simulink model "Active_Suspension_Control_Simulink"  (R2023b)
settings: Solver=VariableStepAuto  StartTime=0.0  StopTime=10.0  MaxStep=1e-3  RelTol=1e-3
values from neighbouring files (symbols this model uses):
  a = [1 20 3486.66666667 10555.5555556 168888.888889]    [Fuzzy_Workspace.mat]    (also in quarter_car_model.m = 0.8)
  b = [0 0 0.00333333333333 10555.6111112 168900.333335]    [Fuzzy_Workspace.mat]
  c_car = 1000    [Active_Suspension_Control.m]    (also in Fuzzy_Workspace.mat)
  k_car = 16000    [Active_Suspension_Control.m]    (also in Fuzzy_Workspace.mat)
  k_wheel = 190000    [Active_Suspension_Control.m]    (also in Fuzzy_Workspace.mat)
  m_car = 300    [Active_Suspension_Control.m]    (also in Fuzzy_Workspace.mat)
  m_wheel = 60    [Active_Suspension_Control.m]    (also in Fuzzy_Workspace.mat)
libraries: slpidlib x1
settings Model: Creator=hkurt  LastModifiedBy=hkurt

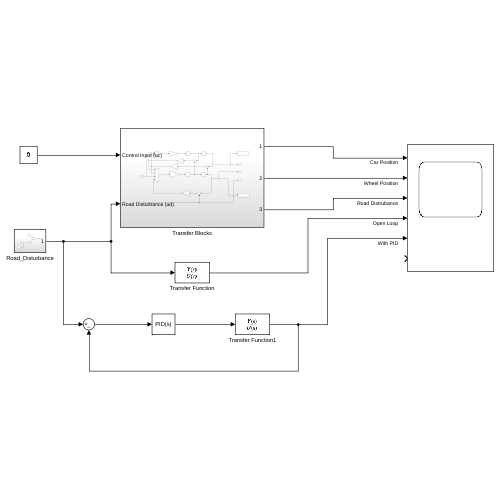
[thumbnail: Simulink's stored preview of the top-level diagram]
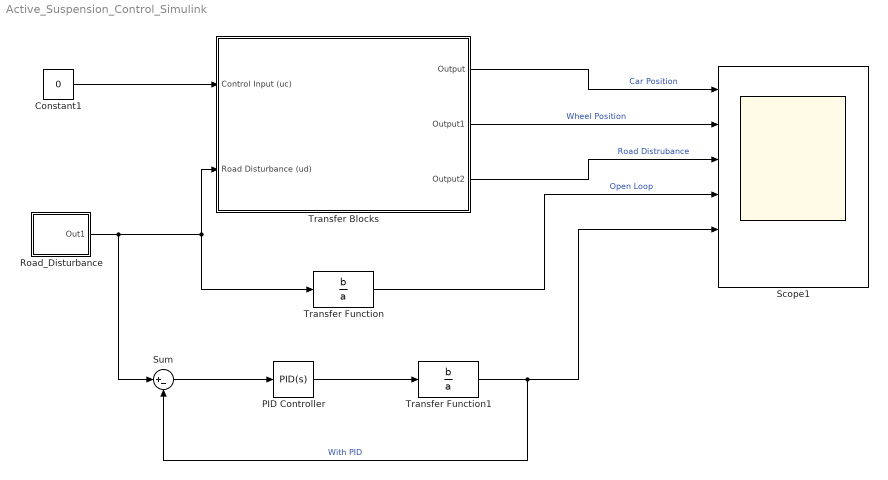
== system Active_Suspension_Control_Simulink ==
  Constant1 : Constant  Value=0
  PID Controller : slpidlib/PID Controller  Controller=PID  Form=Parallel  TimeDomain=Continuous-time  UseExternalTs=off  SampleTime=-1  IntegratorMethod=Forward Euler  FilterMethod=Forward Euler  ControllerParametersSource=internal  P=1  I=10  UseKiTs=off  D=0  N=100  UseFilter=on  TunerSelectOption=Transfer Function Based (PID Tuner App)  InitialConditionSource=internal  InitialConditionForIntegrator=0  InitialConditionForFilter=0  DifferentiatorICPrevScaledInput=0  ExternalReset=none  TrackingMode=off  Kt=1  LimitOutput=off  SatLimitsSource=internal  UpperSaturationLimit=inf  LowerSaturationLimit=-inf  LinearizeAsGain=on  AntiWindupMode=none  Kb=1  LimitIntegrator=off  UpperIntegratorSaturationLimit=inf  LowerIntegratorSaturationLimit=-inf  POutMin=[]  POutMax=[]  IOutMin=[]  IOutMax=[]  DOutMin=[]  DOutMax=[]  NOutMin=[]  NOutMax=[]  SumOutMin=[]  SumOutMax=[]  SaturationOutMin=[]  SaturationOutMax=[]  PParamMin=[]  PParamMax=[]  IParamMin=[]  IParamMax=[]  DParamMin=[]  DParamMax=[]  NParamMin=[]  NParamMax=[]  KbParamMin=[]  KbParamMax=[]  KtParamMin=[]  KtParamMax=[]  KbOutMin=[]  KbOutMax=[]  KtOutMin=[]  KtOutMax=[]  IntegratorOutMin=[]  IntegratorOutMax=[]  FilterOutMin=[]  FilterOutMax=[]  SumI1OutMin=[]  SumI1OutMax=[]  SumI2OutMin=[]  SumI2OutMax=[]  SumI3OutMin=[]  SumI3OutMax=[]  SumI4OutMin=[]  SumI4OutMax=[]  SumDOutMin=[]  SumDOutMax=[]  DifferentiatorOutMin=[]  DifferentiatorOutMax=[]  FilterDiffOutCoefMin=[]  FilterDiffOutCoefMax=[]  ReciprocalOutMin=[]  ReciprocalOutMax=[]  SumDenOutMin=[]  SumDenOutMax=[]  SumNumOutMin=[]  SumNumOutMax=[]  DivideOutMin=[]  DivideOutMax=[]  UdiffTsProdOutMin=[]  UdiffTsProdOutMax=[]  NTsProdOutMin=[]  NTsProdOutMax=[]  UintegralTsProdOutMin=[]  UintegralTsProdOutMax=[]  UngainTsProdOutMin=[]  UngainTsProdOutMax=[]  ClampingZeroOutDataTypeStr=Inherit: Inherit via back propagation  ClampingZeroOutMin=[]  ClampingZeroOutMax=[]  FilterDenConstantOutDataTypeStr=Inherit: Inherit via back propagation  FilterDenConstantOutMin=[]  FilterDenConstantOutMax=[]  PCopyOutDataTypeStr=Inherit: Inherit via back propagation  PCopyOutMin=[]  PCopyOutMax=[]  NCopyOutDataTypeStr=Inherit: Inherit via back propagation  NCopyOutMin=[]  NCopyOutMax=[]  IntegratorContinuousStateAttributes=''  IntegratorStateMustResolveToSignalObject=off  IntegratorRTWStateStorageClass=Auto  FilterContinuousStateAttributes=''  FilterStateMustResolveToSignalObject=off  FilterRTWStateStorageClass=Auto  ParallelPVariant=InternalParameters  IdealPVariant=Disabled  IVariant=InternalParameters  DVariant=InternalParameters  IntegratorVariant=Continuous  SatVariant=Disabled  AWVariant=Passthrough  PCopyVariant=Disabled  TRVariant=Disabled  FdbkBlocksVariant=Forward  IdealPFdbkVariant=Disabled  SatFdbkVariant=Disabled  DerivativeFilterVariant=ContFilter  NVariant=InternalParameters  NCopyVariant=Disabled  FilterICVariant=InternalICsFilter  IntegratorICVariant=InternalICs  ExternalResetVariant=Disabled  TRSumVariant=Passthrough  SumFdbkVariant=Disabled  SumVariant=Sum_PID  TsampFilterVariant=InternalTs  TsampNgainVariant=Passthrough  TsampIntegralVariant=Disabled_SignalSpec  ExternalSaturationOutDataTypeStr=Inherit: Same as second input
  Road_Disturbance : Subsystem
  Scope1 : Scope  NumInputPorts=6
  Sum : Sum  Inputs=|+-
  Transfer Blocks : Subsystem
  Transfer Function : TransferFcn  Numerator=b  Denominator=a
  Transfer Function1 : TransferFcn  Numerator=b  Denominator=a
  wires:
  Transfer Blocks/2(Output1) -> Scope1/2  "Wheel Position"
  Transfer Blocks/3(Output2) -> Scope1/3  "Road Distrubance"
  Constant1/1 -> Transfer Blocks/1(Control Input (uc))
  Transfer Blocks/1(Output) -> Scope1/1  "Car Position"
  Road_Disturbance/1(Out1) -> Sum/1, Transfer Function/1, Transfer Blocks/2(Road Disturbance (ud))
  Transfer Function/1 -> Scope1/4  "Open Loop"
  PID Controller/1 -> Transfer Function1/1
  Transfer Function1/1 -> Scope1/5, Sum/2  "With PID"
  Sum/1 -> PID Controller/1

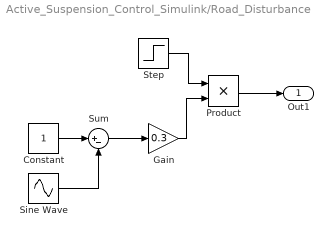
== system Active_Suspension_Control_Simulink/Road_Disturbance ==
  Constant : Constant
  Gain : Gain  Gain=0.3
  Product : Product
  Sine Wave : Sin  Frequency=2*pi  Phase=pi/2  SampleTime=0
  Step : Step  Before=1  After=0  SampleTime=0
  Sum : Sum  Inputs=|+-
  Out1 : Outport
  wires:
  Constant/1 -> Sum/1
  Step/1 -> Product/1
  Sum/1 -> Gain/1
  Gain/1 -> Product/2
  Product/1 -> Out1/1
  Sine Wave/1 -> Sum/2

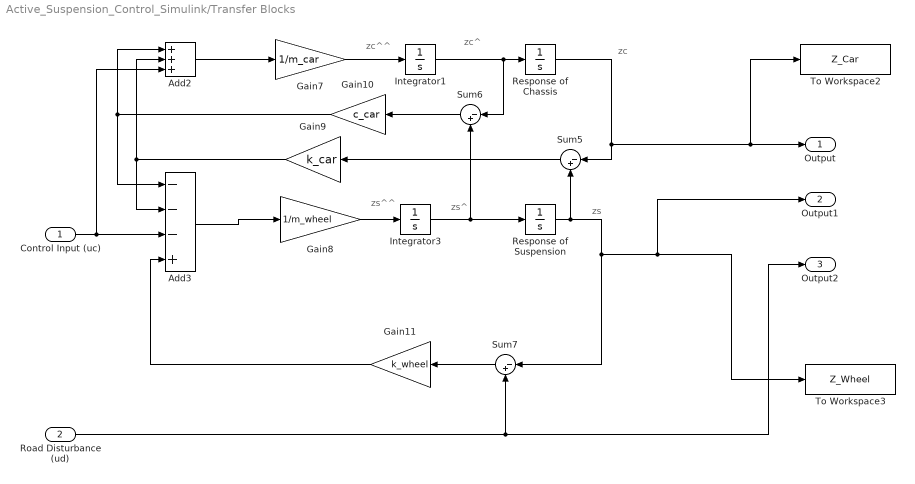
== system Active_Suspension_Control_Simulink/Transfer Blocks ==
  note: zs
  note: zc^^
  note: zc
  note: zc^
  note: zs^^
  note: zs^
  Control Input (uc) : Inport
  Road Disturbance (ud) : Inport  Port=2
  Add2 : Sum  Inputs=+++
  Add3 : Sum  Inputs=---+
  Gain10 : Gain  Gain=c_car
  Gain11 : Gain  Gain=k_wheel
  Gain7 : Gain  Gain=1/m_car
  Gain8 : Gain  Gain=1/m_wheel
  Gain9 : Gain  Gain=k_car
  Integrator1 : Integrator
  Integrator3 : Integrator
  Response of Chassis : Integrator
  Response of Suspension : Integrator
  Sum5 : Sum  Inputs=|-+
  Sum6 : Sum  Inputs=|-+
  Sum7 : Sum  Inputs=|-+
  To Workspace2 : ToWorkspace  VariableName=Z_Car  SaveFormat=Timeseries  SampleTime=-1
  To Workspace3 : ToWorkspace  VariableName=Z_Wheel  SaveFormat=Timeseries  SampleTime=-1
  Output : Outport
  Output1 : Outport  Port=2
  Output2 : Outport  Port=3
  wires:
  Gain11/1 -> Add3/4
  Sum5/1 -> Gain9/1
  Add3/1 -> Gain8/1
  Response of Suspension/1 -> Sum5/2, Sum7/1, Output1/1, To Workspace3/1
  Sum7/1 -> Gain11/1
  Integrator1/1 -> Sum6/1, Response of Chassis/1
  Gain8/1 -> Integrator3/1
  Gain9/1 -> Add3/2, Add2/2
  Sum6/1 -> Gain10/1
  Response of Chassis/1 -> Sum5/1, Output/1, To Workspace2/1
  Gain7/1 -> Integrator1/1
  Road Disturbance (ud)/1 -> Sum7/2, Output2/1
  Integrator3/1 -> Sum6/2, Response of Suspension/1
  Add2/1 -> Gain7/1
  Gain10/1 -> Add3/1, Add2/1
  Control Input (uc)/1 -> Add2/3, Add3/3
